simulink model "ex01_host_disp_image_demo"  (Simulink 7.3)
settings: Solver=ode45  StartTime=0.0  StopTime=inf  RelTol=1e-3
undefined symbols (not defined in the file): gray
libraries: vipsnks x2, dspsigattribs x1, waijung_socket_lib x1
settings Model: Creator=Krisada  LastModifiedBy=Krisada

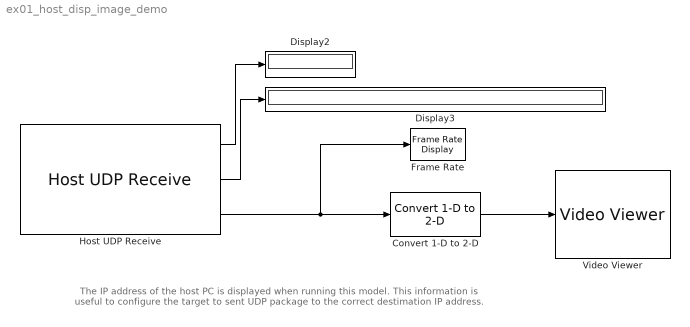
== system ex01_host_disp_image_demo ==
  note: The IP address of the host PC is displayed when running this model.
      | This information is useful to configure the target to sent UDP package to the correct destimation IP address.
  Convert 1-D to 2-D : dspsigattribs/Convert 1-D to 2-D  SystemSampleTime=-1  M=160  N=120  frameBasedOut=off
  Display2 : Display
  Display3 : Display
  Frame Rate : vipsnks/Frame Rate Display  DialogController=vipDDGCreate  DialogControllerArgs=DataTag0  UpdateRate=10
  Host UDP Receive : waijung_socket_lib/Host UDP Receive  conf=HostReceive  protocol=UDP  port=7  address=192.168.1.21  echo=off  transfer=Blocking  timeout=8  datasource=BufferStream  datatype=uint8  datacount=120*160  porttype_double=0  porttype_single=0  porttype_int8=0  porttype_uint8=0  porttype_int16=0  porttype_uint16=0  porttype_int32=0  porttype_uint32=1  portpinstr=0  sampletime=0.1  blockid=HostUDPReceive  inputporttype=[]  inputportwidth=[]  inputportlabel={}  outputporttype=[5,3,3]  outputportwidth=[1,4,19200]  outputportlabel={'Remote Port','Remote IP(1:4)','Data(1:19200)'}  compat=0  optionstring=[]  options=[7,2,1,8000,1]
  Video Viewer : vipsnks/Video Viewer  DialogControllerArgs=DataTag2  inputType=Obsolete7b  imagePorts=One multidimensional signal  useColorMap=off  colormapValue=gray(256)  specRange=off  minInputVal=0  maxInputVal=255  FigPos=[190 518 431 373]  AxisZoom=on  trueSizedOnce=off  OpenAtMdlStart=on
  wires:
  Host UDP Receive/3 -> Frame Rate/1, Convert 1-D to 2-D/1
  Host UDP Receive/1 -> Display2/1
  Host UDP Receive/2 -> Display3/1
  Convert 1-D to 2-D/1 -> Video Viewer/1
